simulink model "stellaris_lp_ls7366r"  (R2017a)
settings: Solver=ode3  StartTime=0.0  StopTime=10.0  FixedStep=0.01  RelTol=1e-3
libraries: stellaris_lp_lib x4
settings Model: ExtModeTrigDuration=2  Creator=peselnikmg  LastModifiedBy=Nilim
settings DataIOCC: LimitDataPoints=on  SaveFormat=Array  SignalLoggingSaveFormat=ModelDataLogs
settings OptimizationCC: PassReuseOutputArgsAs=Individual arguments  ExpressionDepthLimit=2147483647  MaxStackSize=64
settings DebuggingCC: ParameterTunabilityLossMsg=error  StateNameClashWarn=warning  SFUnexpectedBacktrackingDiag=warning  SFNoUnconditionalDefaultTransitionDiag=warning  SFExecutionAtInitializationDiag=none
settings HardwareCC: ProdBitPerPointer=32  ProdBitPerSizeT=32  ProdBitPerPtrDiffT=32  ProdLargestAtomicInteger=Long  ProdLargestAtomicFloat=Double  ProdWordSize=32  ProdHWDeviceType=ARM Compatible->ARM Cortex
settings ModelReferenceCC: PropagateSignalLabelsOutOfModel=off
settings SFSimCC: MATLABDynamicMemAlloc=off
settings RTWCC: SystemTargetFile=ert.tlc  HardwareBoard=Tiva TM4C123G Launchpad  TLCOptions=-aInlineSetEventsForThisBaseRateFcn=TLC_FALSE -aSuppressMultiTaskScheduler=TLC_FALSE -aRateBasedStepFcn=1  TemplateMakefile=ert_default_tmf  Description=Embedded Coder  GenerateReport=on  RTWVerbose=off  Toolchain=Texas Instruments Code Composer Studio (Tiva)  IncludeHyperlinkInReport=on  LaunchReport=on  GenerateTraceInfo=on  GenerateTraceReport=on  GenerateTraceReportSl=on  GenerateTraceReportSf=on  GenerateTraceReportEml=on
settings CodeAppCC: ForceParamTrailComments=on  IgnoreCustomStorageClasses=off  OperatorAnnotations=on  SimulinkDataObjDesc=on  SFDataObjDesc=on  MATLABFcnDesc=on  CustomSymbolStrType=$N$R$M  InsertBlockDesc=on  MATLABSourceComments=on  InternalIdentifier=Classic
settings ConfigComp: CovMetricSettings=dw  CovHtmlReporting=on  CovSaveCumulativeToWorkspaceVar=on  CovSaveSingleToWorkspaceVar=on  CovExternalEMLEnable=off

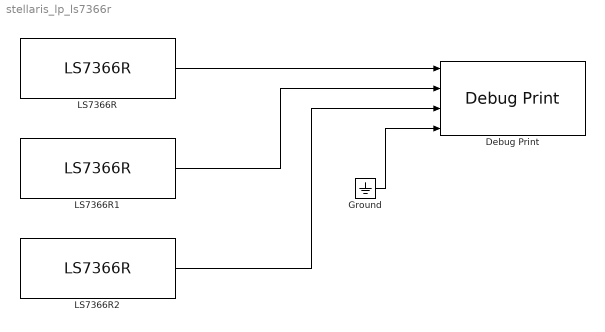
== system stellaris_lp_ls7366r ==
  Debug Print : stellaris_lp_lib/Debug/Debug Print  fmt="'counter =  %d %d %d'"  sample_time=-1
      settings: SourceProductName=Run on Stellaris LaunchPad
  Ground : Ground
  LS7366R : stellaris_lp_lib/SPIDev/LS7366R  ssel="CH 1  (SSEL: PA3)"  ext_clk=on  sample_time=0.01
      settings: SourceProductName=Run on Stellaris LaunchPad
  LS7366R1 : stellaris_lp_lib/SPIDev/LS7366R  ssel="CH 2  (SSEL: PD0)"  ext_clk=on  sample_time=0.01
      settings: SourceProductName=Run on Stellaris LaunchPad
  LS7366R2 : stellaris_lp_lib/SPIDev/LS7366R  ssel="CH 3  (SSEL: PD1)"  ext_clk=on  sample_time=0.01
      settings: SourceProductName=Run on Stellaris LaunchPad
  wires:
  LS7366R/1 -> Debug Print/1
  Ground/1 -> Debug Print/4
  LS7366R1/1 -> Debug Print/2
  LS7366R2/1 -> Debug Print/3
